simulink model "levitacionMagnetica"  (R2021a)
settings: Solver=VariableStepAuto  StartTime=0.0  StopTime=800  RelTol=1e-3
settings Model: Creator=jmata  LastModifiedBy=jmata

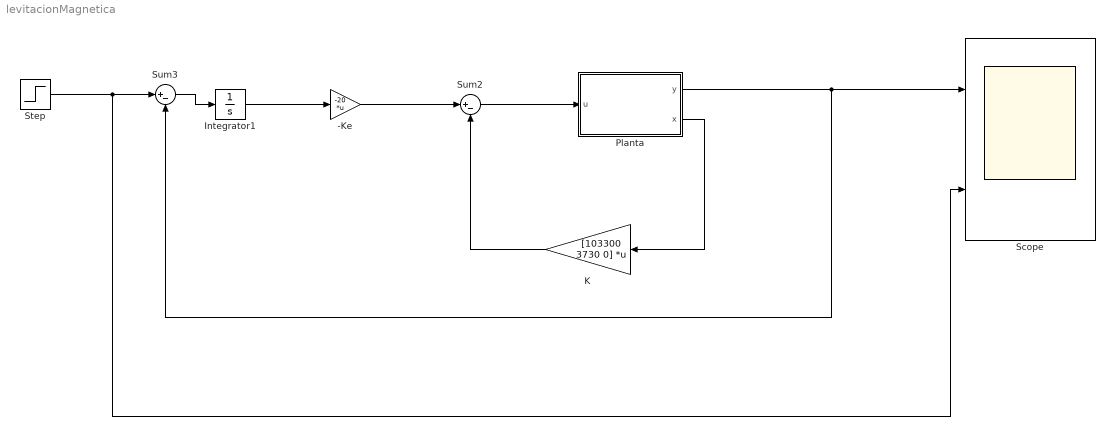
== system levitacionMagnetica ==
  -Ke : Gain  Gain=-20  Multiplication=Matrix(K*u)
  Integrator1 : Integrator
  K : Gain  Gain=[103300 3730 0]  Multiplication=Matrix(K*u)
  Planta : Subsystem
  Scope : Scope  NumInputPorts=2
  Step : Step  SampleTime=0
  Sum2 : Sum  Inputs=|+-
  Sum3 : Sum  Inputs=|+-
  wires:
  Sum3/1 -> Integrator1/1
  -Ke/1 -> Sum2/1
  Planta/2(x) -> K/1
  Planta/1(y) -> Sum3/2, Scope/1
  Step/1 -> Scope/2, Sum3/1
  Sum2/1 -> Planta/1(u)
  Integrator1/1 -> -Ke/1
  K/1 -> Sum2/2

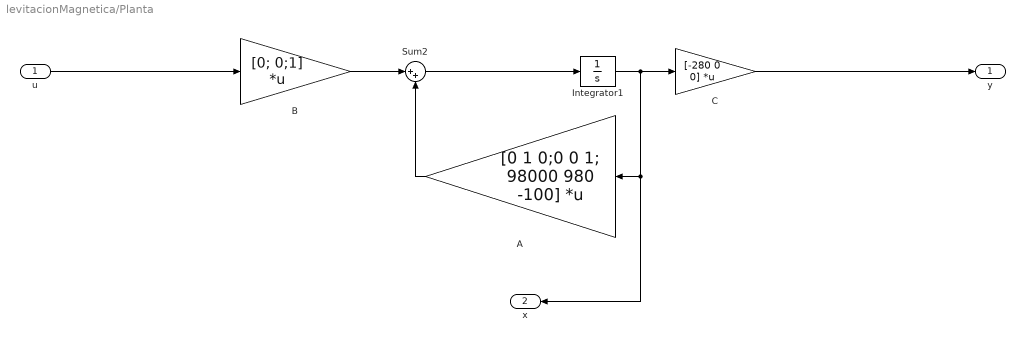
== system levitacionMagnetica/Planta ==
  u : Inport
  A : Gain  Gain=[0 1 0;0 0 1; 98000 980 -100]  Multiplication=Matrix(K*u)
  B : Gain  Gain=[0; 0;1]  Multiplication=Matrix(K*u)
  C : Gain  Gain=[-280 0 0]  Multiplication=Matrix(K*u)
  Integrator1 : Integrator
  Sum2 : Sum  Inputs=|++
  y : Outport
  x : Outport  Port=2
  wires:
  Sum2/1 -> Integrator1/1
  A/1 -> Sum2/2
  Integrator1/1 -> x/1, A/1, C/1
  B/1 -> Sum2/1
  u/1 -> B/1
  C/1 -> y/1
